simulink model "Drone_Sim_New"  (R2022b)
settings: Solver=VariableStepAuto  StartTime=0.0  StopTime=10.0  RelTol=1e-3
libraries: fuzblock x7
settings Model: Creator=frz  LastModifiedBy=frz

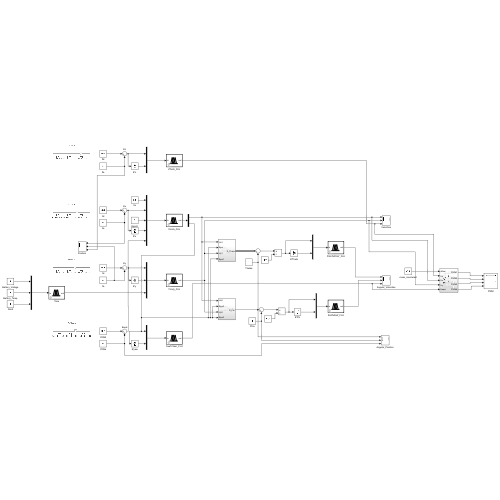
[thumbnail: Simulink's stored preview of the top-level diagram]
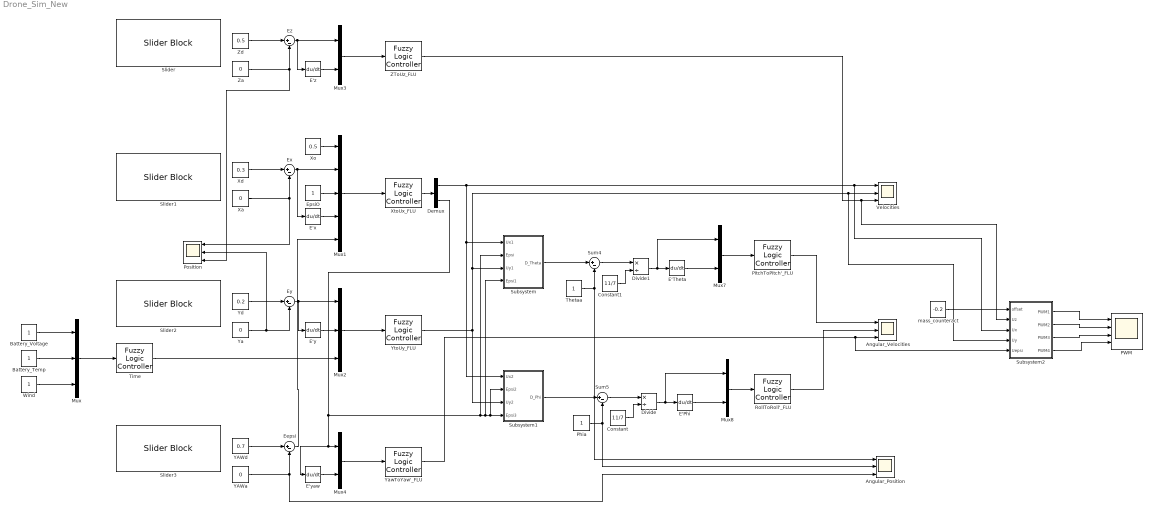
== system Drone_Sim_New ==
  Angular_Position : Scope  NumInputPorts=3
  Angular_Velocities : Scope  NumInputPorts=3
  Battery_Temp : Constant
  Battery_Voltage : Constant
  Constant : Constant  Value=11/7
  Constant1 : Constant  Value=11/7
  Demux : Demux  Outputs=2
  Divide : Product  Inputs=*/
  Divide1 : Product  Inputs=*/
  E'Phi : Derivative
  E'Theta : Derivative
  E'x : Derivative
  E'y : Derivative
  E'yaw : Derivative
  E'z : Derivative
  Eepsi : Sum  Inputs=|+-
  EpsiO : Constant
  Ex : Sum  Inputs=|+-
  Ey : Sum  Inputs=|+-
  Ez : Sum  Inputs=|+-
  Mux : Mux  Inputs=3
  Mux1 : Mux  Inputs=5
  Mux2 : Mux  Inputs=3
  Mux{3..4,7..8} (4 alike) : Mux  Inputs=2
  PWM : Scope  NumInputPorts=4
  Phia : Constant
  PitchToPitch'_FLU : fuzblock/Fuzzy Logic  Controller  FIS='Theta_D.fis'  OutputSampleNumber=101  DataType=double  FuzzifiedInputs=off  RuleFiringStrengths=off  RuleOutputs=off  AggregatedOutputs=off  SimulateUsing=Interpreted execution  OutOfRangeInputValueMessage=warning  NoRuleFiredMessage=warning  EmptyOutputFuzzySetMessage=warning
  Position : Scope  NumInputPorts=3
  RollToRoll'_FLU : fuzblock/Fuzzy Logic  Controller  FIS='Phi_D.fis'  OutputSampleNumber=101  DataType=double  FuzzifiedInputs=off  RuleFiringStrengths=off  RuleOutputs=off  AggregatedOutputs=off  SimulateUsing=Interpreted execution  OutOfRangeInputValueMessage=warning  NoRuleFiredMessage=warning  EmptyOutputFuzzySetMessage=warning
  Slider : SliderBlock  ScaleMin=-1  ScaleMax=1
  Slider1 : SliderBlock  ScaleMin=-1  ScaleMax=1
  Slider2 : SliderBlock  ScaleMin=-1  ScaleMax=1
  Slider3 : SliderBlock  ScaleMin=-3.2  ScaleMax=3.2
  Subsystem : Subsystem
  Subsystem1 : Subsystem
  Subsystem2 : Subsystem
  Sum4 : Sum  Inputs=|+-
  Sum5 : Sum  Inputs=|+-
  Thetaa : Constant
  Time : fuzblock/Fuzzy Logic  Controller  FIS='Time.fis'  OutputSampleNumber=101  DataType=double  FuzzifiedInputs=off  RuleFiringStrengths=off  RuleOutputs=off  AggregatedOutputs=off  SimulateUsing=Interpreted execution  OutOfRangeInputValueMessage=warning  NoRuleFiredMessage=warning  EmptyOutputFuzzySetMessage=warning
  Velocities : Scope  NumInputPorts=3
  Wind : Constant
  Xa : Constant  Value=0
  Xd : Constant  Value=0.3
  Xo : Constant  Value=0.5
  XtoUx_FLU : fuzblock/Fuzzy Logic  Controller  FIS='Ux_EpsiDevX_ObstacleAvoidancefis2.fis'  OutputSampleNumber=101  DataType=double  FuzzifiedInputs=off  RuleFiringStrengths=off  RuleOutputs=off  AggregatedOutputs=off  SimulateUsing=Interpreted execution  OutOfRangeInputValueMessage=warning  NoRuleFiredMessage=warning  EmptyOutputFuzzySetMessage=warning
  YAWa : Constant  Value=0
  YAWd : Constant  Value=0.7
  Ya : Constant  Value=0
  YawToYaw'_FLU : fuzblock/Fuzzy Logic  Controller  FIS='Epsi_D.fis'  OutputSampleNumber=101  DataType=double  FuzzifiedInputs=off  RuleFiringStrengths=off  RuleOutputs=off  AggregatedOutputs=off  SimulateUsing=Interpreted execution  OutOfRangeInputValueMessage=warning  NoRuleFiredMessage=warning  EmptyOutputFuzzySetMessage=warning
  Yd : Constant  Value=0.2
  YtoUy_FLU : fuzblock/Fuzzy Logic  Controller  FIS='Y_FLU.fis'  OutputSampleNumber=101  DataType=double  FuzzifiedInputs=off  RuleFiringStrengths=off  RuleOutputs=off  AggregatedOutputs=off  SimulateUsing=Interpreted execution  OutOfRangeInputValueMessage=warning  NoRuleFiredMessage=warning  EmptyOutputFuzzySetMessage=warning
  ZToUz_FLU : fuzblock/Fuzzy Logic  Controller  FIS='Z_FLU.fis'  OutputSampleNumber=101  DataType=double  FuzzifiedInputs=off  RuleFiringStrengths=off  RuleOutputs=off  AggregatedOutputs=off  SimulateUsing=Interpreted execution  OutOfRangeInputValueMessage=warning  NoRuleFiredMessage=warning  EmptyOutputFuzzySetMessage=warning
  Za : Constant  Value=0
  Zd : Constant  Value=0.5
  mass_counteract : Constant  Value=-0.2
  wires:
  Zd/1 -> Ez/1
  Xd/1 -> Ex/1
  Yd/1 -> Ey/1
  YAWd/1 -> Eepsi/1
  E'z/1 -> Mux3/2
  E'y/1 -> Mux2/2
  E'yaw/1 -> Mux4/2
  Mux2/1 -> YtoUy_FLU/1
  Mux4/1 -> YawToYaw'_FLU/1
  Mux1/1 -> XtoUx_FLU/1
  Mux3/1 -> ZToUz_FLU/1
  Mux7/1 -> PitchToPitch'_FLU/1
  E'Theta/1 -> Mux7/2
  E'Phi/1 -> Mux8/2
  Mux8/1 -> RollToRoll'_FLU/1
  Za/1 -> Position/3, Ez/2
  Xa/1 -> Position/1, Ex/2
  Ya/1 -> Ey/2, Position/2
  YAWa/1 -> Angular_Position/3, Eepsi/2
  Thetaa/1 -> Angular_Position/1, Sum4/2
  Ez/1 -> E'z/1, Mux3/1
  Ex/1 -> Mux1/2, E'x/1
  Ey/1 -> E'y/1, Mux2/1
  Mux/1 -> Time/1
  Battery_Voltage/1 -> Mux/1
  Battery_Temp/1 -> Mux/2
  Wind/1 -> Mux/3
  Time/1 -> Mux2/3
  XtoUx_FLU/1 -> Demux/1
  YtoUy_FLU/1 -> Subsystem2/4(Uy), Velocities/2, Subsystem/3(Uy1), Subsystem1/3(Uy2)
  Subsystem/1(D_Theta) -> Sum4/1
  Subsystem1/1(D_Phi) -> Sum5/1
  RollToRoll'_FLU/1 -> Angular_Velocities/2
  PitchToPitch'_FLU/1 -> Angular_Velocities/1
  ZToUz_FLU/1 -> Subsystem2/2(Uz), Velocities/3
  Phia/1 -> Angular_Position/2, Sum5/2
  Xo/1 -> Mux1/1
  EpsiO/1 -> Mux1/3
  E'x/1 -> Mux1/4
  Demux/1 -> Subsystem1/1(Ux2), Subsystem/1(Ux1), Subsystem2/3(Ux), Velocities/1
  Eepsi/1 -> Mux1/5
  YawToYaw'_FLU/1 -> Subsystem2/5(Uepsi), Angular_Velocities/3
  Demux/2 -> Subsystem/2(Epsi), Subsystem/4(Epsi1), Subsystem1/2(Epsi2), Subsystem1/4(Epsi3), E'yaw/1, Mux4/1
  Subsystem2/1(PWM1) -> PWM/1
  Subsystem2/2(PWM2) -> PWM/2
  Subsystem2/3(PWM3) -> PWM/3
  Subsystem2/4(PWM4) -> PWM/4
  Divide/1 -> Mux8/1, E'Phi/1
  Sum5/1 -> Divide/1
  Constant/1 -> Divide/2
  Constant1/1 -> Divide1/2
  Sum4/1 -> Divide1/1
  Divide1/1 -> Mux7/1, E'Theta/1
  mass_counteract/1 -> Subsystem2/1(offset)

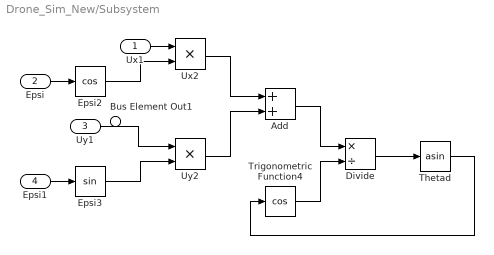
== system Drone_Sim_New/Subsystem ==
  Ux1 : Inport
  Epsi : Inport  Port=2
  Uy1 : Inport  Port=3
  Epsi1 : Inport  Port=4
  Add : Sum
  Divide : Product  Inputs=*/
  Epsi2 : Trigonometry  Operator=cos
  Epsi3 : Trigonometry
  Thetad : Trigonometry  Operator=asin
  Trigonometric Function4 : Trigonometry  Operator=cos
  Ux2 : Product
  Uy2 : Product
  Bus Element Out1 : Outport  PortName=D_Theta  Element=signal1
  wires:
  Epsi2/1 -> Ux2/2
  Divide/1 -> Thetad/1
  Thetad/1 -> Trigonometric Function4/1
  Add/1 -> Divide/1
  Epsi3/1 -> Uy2/2
  Ux2/1 -> Add/1
  Uy2/1 -> Add/2
  Trigonometric Function4/1 -> Divide/2
  Uy1/1 -> Uy2/1
  Ux1/1 -> Ux2/1
  Epsi1/1 -> Epsi3/1
  Epsi/1 -> Epsi2/1

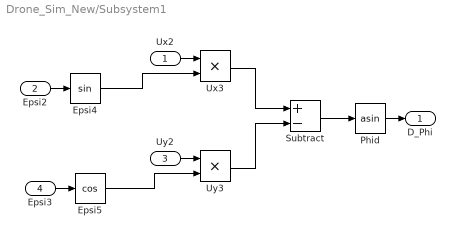
== system Drone_Sim_New/Subsystem1 ==
  Ux2 : Inport
  Epsi2 : Inport  Port=2
  Uy2 : Inport  Port=3
  Epsi3 : Inport  Port=4
  Epsi4 : Trigonometry
  Epsi5 : Trigonometry  Operator=cos
  Phid : Trigonometry  Operator=asin
  Subtract : Sum  Inputs=+-
  Ux3 : Product
  Uy3 : Product
  D_Phi : Outport
  wires:
  Epsi3/1 -> Epsi5/1
  Ux3/1 -> Subtract/1
  Epsi5/1 -> Uy3/2
  Subtract/1 -> Phid/1
  Uy2/1 -> Uy3/1
  Uy3/1 -> Subtract/2
  Epsi4/1 -> Ux3/2
  Epsi2/1 -> Epsi4/1
  Phid/1 -> D_Phi/1
  Ux2/1 -> Ux3/1

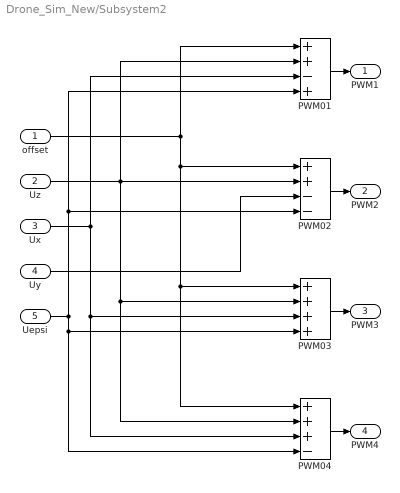
== system Drone_Sim_New/Subsystem2 ==
  offset : Inport
  Uz : Inport  Port=2
  Ux : Inport  Port=3
  Uy : Inport  Port=4
  Uepsi : Inport  Port=5
  PWM01 : Sum  Inputs=++-+
  PWM02 : Sum  Inputs=++--
  PWM03 : Sum  Inputs=++++
  PWM04 : Sum  Inputs=+++-
  PWM1 : Outport
  PWM2 : Outport  Port=2
  PWM3 : Outport  Port=3
  PWM4 : Outport  Port=4
  wires:
  offset/1 -> PWM04/1, PWM03/1, PWM02/1, PWM01/1
  Uepsi/1 -> PWM04/4, PWM03/4, PWM01/4, PWM02/4
  Ux/1 -> PWM04/3, PWM03/3, PWM01/3
  Uz/1 -> PWM04/2, PWM03/2, PWM02/2, PWM01/2
  PWM02/1 -> PWM2/1
  Uy/1 -> PWM02/3
  PWM03/1 -> PWM3/1
  PWM01/1 -> PWM1/1
  PWM04/1 -> PWM4/1
